simulink model "TACHOMETER"  (R2019b)
settings: Solver=VariableStepAuto  StartTime=0.0  StopTime=10.0  RelTol=1e-3
undefined symbols (not defined in the file): coil_mass, magnet_flux, timeStep
libraries: simulink_extras x2, eeGeneralControl x1
settings Model: Creator=simone  LastModifiedBy=simone

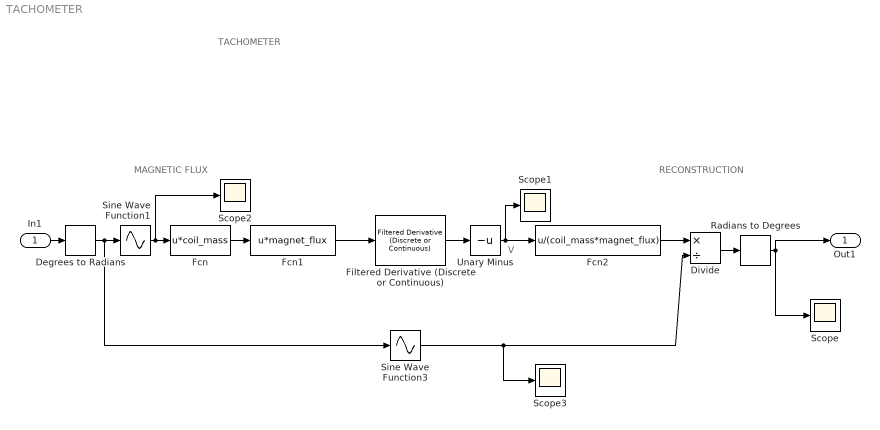
== system TACHOMETER ==
  note: RECONSTRUCTION
  note: TACHOMETER
  note: V
  note: MAGNETIC FLUX
  In1 : Inport
  Degrees to Radians : simulink_extras/Transformations/Degrees to Radians
  Divide : Product  Inputs=*/
  Fcn : Fcn  Expr=u*coil_mass
  Fcn1 : Fcn  Expr=u*magnet_flux
  Fcn2 : Fcn  Expr=u/(coil_mass*magnet_flux)
  Filtered Derivative (Discrete or Continuous) : eeGeneralControl/Filtered Derivative (Discrete or Continuous)  K=1  T=0  B=inf  A=-inf  minRatio=1  Ts=timeStep
      settings: SourceProductName=Simscape Electrical  SourceProductBaseCode=PS
  Radians to Degrees : simulink_extras/Transformations/Radians to Degrees
  Scope{,1..3} (4 alike) : Scope
  Sine Wave Function1 : Sin  TimeSource=Use external signal  Phase=pi/2  SampleTime=0
  Sine Wave Function3 : Sin  TimeSource=Use external signal  SampleTime=0
  Unary Minus : UnaryMinus
  Out1 : Outport
  wires:
  Sine Wave Function1/1 -> Scope2/1, Fcn/1
  Fcn/1 -> Fcn1/1
  Unary Minus/1 -> Scope1/1, Fcn2/1
  Fcn2/1 -> Divide/1
  Divide/1 -> Radians to Degrees/1
  In1/1 -> Degrees to Radians/1
  Degrees to Radians/1 -> Sine Wave Function3/1, Sine Wave Function1/1
  Radians to Degrees/1 -> Scope/1, Out1/1
  Fcn1/1 -> Filtered Derivative (Discrete or Continuous)/1
  Filtered Derivative (Discrete or Continuous)/1 -> Unary Minus/1
  Sine Wave Function3/1 -> Scope3/1, Divide/2
